simulink model "sim_cascade_model"  (R2024a)
settings: Solver=ode4  StartTime=0.0  StopTime=500  FixedStep=0.02  RelTol=1e-3
undefined symbols (not defined in the file or in its folder): Ki1, Ki2, Kp1, Kp2, p, r_ref, t_ref
settings Model: Creator=marius  LastModifiedBy=marius

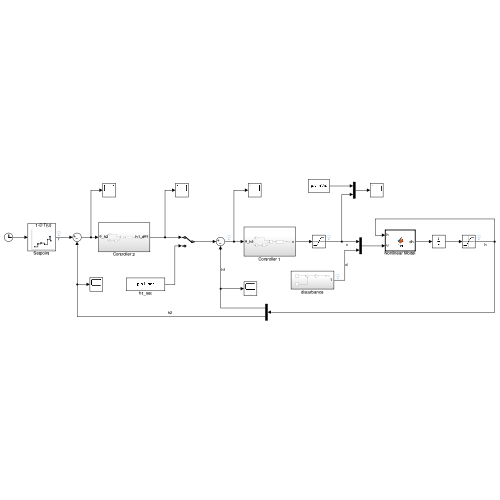
[thumbnail: Simulink's stored preview of the top-level diagram]
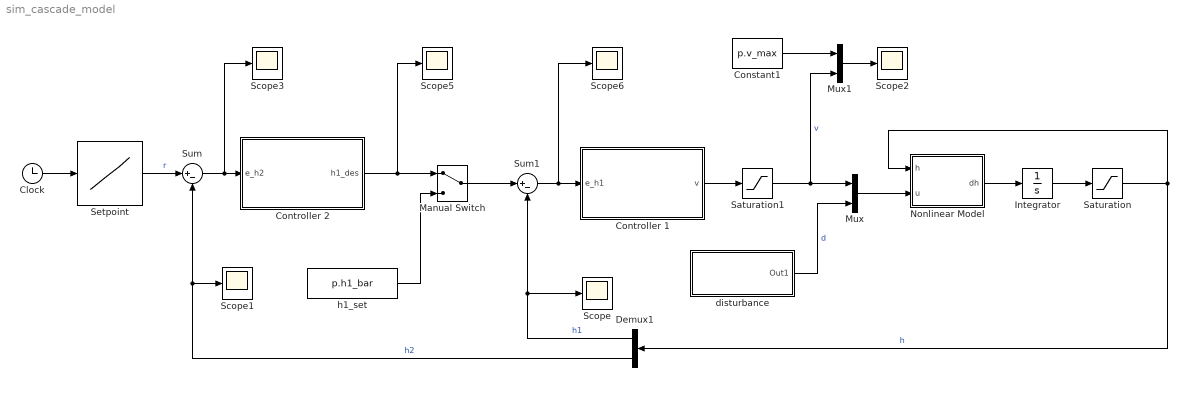
== system sim_cascade_model ==
  Clock : Clock
  Constant1 : Constant  Value=p.v_max
  Controller 1 : Subsystem
  Controller 2 : Subsystem
  Demux1 : Demux  Outputs=2
  Integrator : Integrator  InitialCondition=[p.h1_bar; p.h2_bar]
  Manual Switch : ManualSwitch
  Mux : Mux  Inputs=2
  Mux1 : Mux  Inputs=2
  Nonlinear Model : MATLAB Function  TreatAsAtomicUnit=on
  Saturation : Saturate  UpperLimit=p.h_max  LowerLimit=0
  Saturation1 : Saturate  UpperLimit=p.v_max  LowerLimit=0
  Scope{,1..3,5..6} (6 alike) : Scope
  Setpoint : Lookup_n-D  NumberOfTableDimensions=1  BreakpointsForDimension1=t_ref  Table=r_ref  InterpMethod=Flat  InternalRulePriority=Speed  RndMeth=Simplest
  Sum : Sum  Inputs=|+-
  Sum1 : Sum  Inputs=|+-
  disturbance : Subsystem
  h1_set : Constant  Value=p.h1_bar
  wires:
  Nonlinear Model/1(dh) -> Integrator/1
  Integrator/1 -> Saturation/1
  Mux/1 -> Nonlinear Model/2(u)
  Sum/1 -> Controller 2/1(e_h2), Scope3/1
  Setpoint/1 -> Sum/1  "r"
  disturbance/1(Out1) -> Mux/2  "d"
  Saturation/1 -> Nonlinear Model/1(h), Demux1/1  "h"
  Saturation1/1 -> Mux/1, Mux1/2  "v"
  Demux1/1 -> Scope/1, Sum1/2  "h1"
  Demux1/2 -> Scope1/1, Sum/2  "h2"
  Sum1/1 -> Scope6/1, Controller 1/1(e_h1)
  Manual Switch/1 -> Sum1/1
  Controller 2/1(h1_des) -> Scope5/1, Manual Switch/1
  h1_set/1 -> Manual Switch/2
  Mux1/1 -> Scope2/1
  Constant1/1 -> Mux1/1
  Controller 1/1(v) -> Saturation1/1
  Clock/1 -> Setpoint/1

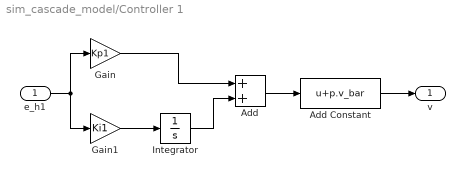
== system sim_cascade_model/Controller 1 ==
  e_h1 : Inport
  Add : Sum
  Add Constant : Bias  Bias=p.v_bar  SaturateOnIntegerOverflow=off
  Gain : Gain  Gain=Kp1
  Gain1 : Gain  Gain=Ki1
  Integrator : Integrator
  v : Outport
  wires:
  e_h1/1 -> Gain1/1, Gain/1
  Gain1/1 -> Integrator/1
  Integrator/1 -> Add/2
  Gain/1 -> Add/1
  Add/1 -> Add Constant/1
  Add Constant/1 -> v/1

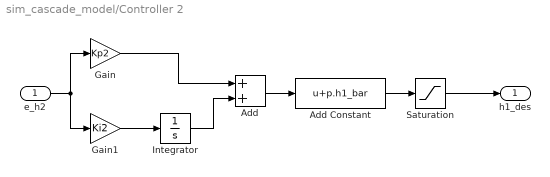
== system sim_cascade_model/Controller 2 ==
  e_h2 : Inport
  Add : Sum
  Add Constant : Bias  Bias=p.h1_bar  SaturateOnIntegerOverflow=off
  Gain : Gain  Gain=Kp2
  Gain1 : Gain  Gain=Ki2
  Integrator : Integrator
  Saturation : Saturate  UpperLimit=p.h_max  LowerLimit=0
  h1_des : Outport
  wires:
  e_h2/1 -> Gain1/1, Gain/1
  Gain1/1 -> Integrator/1
  Integrator/1 -> Add/2
  Gain/1 -> Add/1
  Add/1 -> Add Constant/1
  Add Constant/1 -> Saturation/1
  Saturation/1 -> h1_des/1

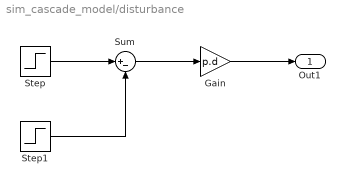
== system sim_cascade_model/disturbance ==
  Gain : Gain  Gain=p.d
  Step : Step  Time=p.dt_on  SampleTime=0
  Step1 : Step  Time=p.dt_off  SampleTime=0
  Sum : Sum  Inputs=|+-
  Out1 : Outport
  wires:
  Step/1 -> Sum/1
  Sum/1 -> Gain/1
  Step1/1 -> Sum/2
  Gain/1 -> Out1/1

== matlab function sim_cascade_model/Nonlinear Model ==
  data: h input; u input; dh output; p parameter
function dh = fcn(h, u, p)
    [dh, y] = nonlinear_model(h, u, p);
end
